simulink library "pathFollowingExp_LAS"  (R2020a)
settings: Solver=VariableStepAuto  StartTime=0.0  StopTime=10.0  RelTol=1e-3
undefined symbols (not defined in the file or in its folder): fltCtrl, pathCtrl, vhcl
libraries: pathFollowingControllerExp_cl x4, courseFollowExp_cl x1, ctrlAllocMatrix_cl x1
settings Model: Creator=jcreed2  LastModifiedBy=jcreed2

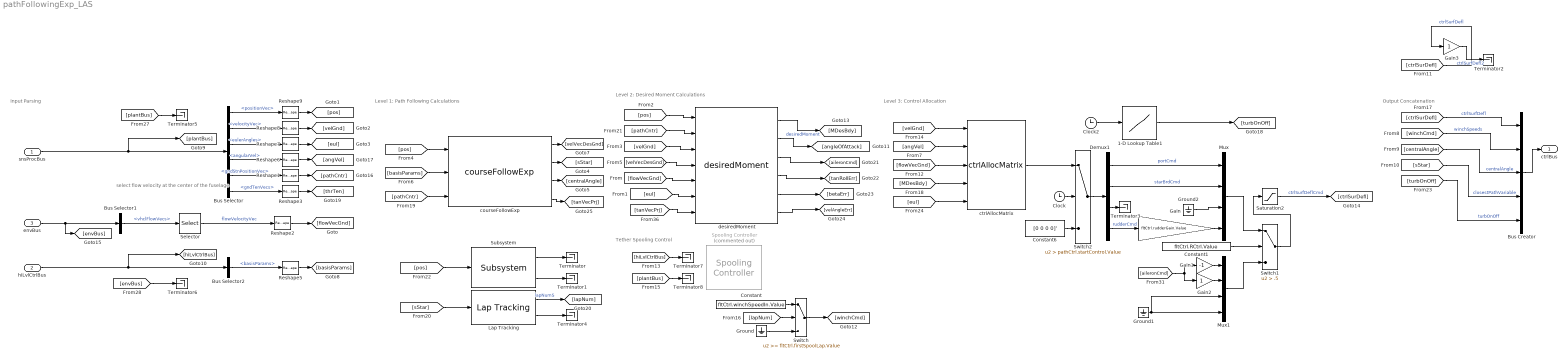
== system pathFollowingExp_LAS ==
  note: Output Concatenation
  note: Level 2: Desired Moment Calculations
  note: Input Parsing
  note: Level 1: Path Following Calculations
  note: Tether Spooling Control
  note: select flow velocity at the center of the fuselage
  note: Level 3: Control Allocation
  snsProcBus : Inport  OutDataTypeStr=Bus: sensorsProcessingBus
  hiLvlCtrlBus : Inport  Port=2  OutDataTypeStr=Bus: hiLvlCtrlBus
  envBus : Inport  Port=3  OutDataTypeStr=Bus: envBus
  1-D Lookup Table1 : Lookup_n-D  NumberOfTableDimensions=1  BreakpointsForDimension1=[0 1000 2000]  Table=[0 0 0]  InterpMethod=Flat  InternalRulePriority=Speed  RndMeth=Simplest  InputSameDT=on
  Bus Creator : BusCreator  Inputs=5  OutDataTypeStr=Bus: fltCtrlBus
      settings: InheritFromInputs=off
  Bus Selector : BusSelector  OutputSignals=positionVec,velocityVec,eulerAngles,angularVel,gndStnPositionVec,gndTenVecs
  Bus Selector1 : BusSelector  OutputSignals=vhclFlowVecs
  Bus Selector2 : BusSelector  OutputSignals=basisParams
  Clock : Clock
  Clock2 : Clock
  Constant : Constant  Value=fltCtrl.winchSpeedIn.Value
  Constant1 : Constant  Value=fltCtrl.RCtrl.Value
  Constant6 : Constant  Value=[0 0 0 0]'
  Demux1 : Demux
  Gain : Gain  Gain=fltCtrl.rudderGain.Value
  Gain1 : Gain  Gain=-1
  Gain2 : Gain
  Gain3 : Gain
  Ground : Ground
  Ground1 : Ground
  Ground2 : Ground
  Lap Tracking : pathFollowingControllerExp_cl/pathFollowingControllerExp/Lap Tracking  SystemSampleTime=-1  Latency=0  AutoFrameSizeCalculation=off
  Mux : Mux
  Mux1 : Mux
  Reshape{1..3,5..9} (8 alike) : Reshape  OutputDimensionality=Column vector (2-D)
  Saturation2 : Saturate  UpperLimit=pathCtrl.controlSigMax.upperLimit.Value  LowerLimit=pathCtrl.controlSigMax.lowerLimit.Value
  Selector : Selector  NumberOfDimensions=2  InputPortWidth=3  IndexOptions=Select all,Index vector (dialog)  Indices=[1 3],5  OutputSizes=1,1
  "Spooling Controller " : pathFollowingControllerExp_cl/pathFollowingControllerExp/Spooling Controller   Commented=on  SystemSampleTime=-1  Latency=0  AutoFrameSizeCalculation=off
  Subsystem : pathFollowingControllerExp_cl/pathFollowingControllerExp/Subsystem  SystemSampleTime=-1  Latency=0  AutoFrameSizeCalculation=off
  Switch : Switch  Threshold=fltCtrl.firstSpoolLap.Value
  Switch1 : Switch  Criteria=u2 > Threshold  Threshold=.5
  Switch2 : Switch  Criteria=u2 > Threshold  Threshold=pathCtrl.startControl.Value
  Terminator{,1..8} (9 alike) : Terminator
  courseFollowExp : courseFollowExp_cl/courseFollowExp  SystemSampleTime=-1  Latency=0  AutoFrameSizeCalculation=off
  ctrlAllocMatrix : ctrlAllocMatrix_cl/ctrlAllocMatrix  aeroStruct=vhcl.struct('OCT.aeroSurf')  fluidDensity=fluidDensity
  desiredMoment : pathFollowingControllerExp_cl/pathFollowingControllerExp/desiredMoment  SystemSampleTime=-1  Latency=0  AutoFrameSizeCalculation=off
  ctrlBus : Outport  OutDataTypeStr=Bus: fltCtrlBus  VectorParamsAs1DForOutWhenUnconnected=off
  wires:
  Bus Selector/6 -> Reshape3/1  "<gndTenVecs>"
  snsProcBus/1 -> [plantBus], Bus Selector/1
  Demux1/1 -> Mux/1  "portCmd"
  [pos] -> courseFollowExp/1
  Demux1/2 -> Mux/2  "starBrdCmd"
  hiLvlCtrlBus/1 -> Bus Selector2/1, [hiLvlCtrlBus]
  Saturation2/1 -> [ctrlSurDefl]  "ctrlSurfDeflCmd"
  Constant/1 -> Switch/1
  Switch1/1 -> Saturation2/1
  courseFollowExp/3 -> [centralAngle]
  Bus Selector/2 -> Reshape8/1  "<velocityVec>"
  [velGnd] -> ctrlAllocMatrix/1
  Bus Selector/3 -> Reshape7/1  "<eulerAngles>"
  Bus Selector1/1 -> Selector/1  "<vhclFlowVecs>"
  Bus Selector/1 -> Reshape9/1  "<positionVec>"
  Lap Tracking/2 -> Terminator4/1
  [pos] -> desiredMoment/1
  Reshape3/1 -> [thrTen]
  envBus/1 -> Bus Selector1/1, [envBus]
  courseFollowExp/1 -> [velVecDesGnd]
  Demux1/4 -> Gain/1  "rudderCmd"
  Bus Creator/1 -> ctrlBus/1
  [winchCmd] -> Bus Creator/2  "winchSpeeds"
  [turbOnOff] -> Bus Creator/5  "turbOnOff"
  courseFollowExp/4 -> [tanVecPrj]
  courseFollowExp/2 -> [sStar]
  Selector/1 -> Reshape2/1  "flowVelocityVec"
  [centralAngle] -> Bus Creator/3  "centralAngle"
  desiredMoment/1 -> [MDesBdy]  "desiredMoment"
  [tanVecPrj] -> desiredMoment/7
  [sStar] -> Bus Creator/4  "closestPathVariable"
  [flowVecGnd] -> ctrlAllocMatrix/3
  [eul] -> desiredMoment/6
  [ctrlSurDefl] -> Gain3/1  "ctrlSurfDefl"
  [ctrlSurDefl] -> Bus Creator/1  "ctrlSurfDefl"
  [pathCntr] -> courseFollowExp/3
  [MDesBdy] -> ctrlAllocMatrix/4
  Constant6/1 -> Switch2/3
  Bus Selector/4 -> Reshape6/1  "<angularVel>"
  Switch2/1 -> Demux1/1
  Reshape6/1 -> [angVel]
  Bus Selector/5 -> Reshape1/1  "<gndStnPositionVec>"
  [pathCntr] -> desiredMoment/2
  Constant1/1 -> Switch1/2
  [flowVecGnd] -> desiredMoment/5
  ctrlAllocMatrix/1 -> Switch2/1
  Reshape2/1 -> [flowVecGnd]
  Reshape8/1 -> [velGnd]
  Reshape1/1 -> [pathCntr]
  [velGnd] -> desiredMoment/3
  Clock2/1 -> 1-D Lookup Table1/1
  [eul] -> ctrlAllocMatrix/5
  Bus Selector2/1 -> Reshape5/1  "<basisParams>"
  Gain/1 -> Mux/4
  [basisParams] -> courseFollowExp/2
  [pos] -> Subsystem/1
  Reshape9/1 -> [pos]
  desiredMoment/2 -> [angleOfAttack]
  Ground2/1 -> Mux/3
  [plantBus] -> Terminator8/1
  Demux1/3 -> Terminator3/1
  Clock/1 -> Switch2/2
  [plantBus] -> Terminator5/1
  Lap Tracking/1 -> [lapNum]  "lapNumS"
  [hiLvlCtrlBus] -> Terminator7/1
  Reshape7/1 -> [eul]
  Subsystem/1 -> Terminator/1
  Subsystem/2 -> Terminator1/1
  [envBus] -> Terminator6/1
  [sStar] -> Lap Tracking/1
  [velVecDesGnd] -> desiredMoment/4
  desiredMoment/3 -> [aileronCmd]
  [angVel] -> ctrlAllocMatrix/2
  [aileronCmd] -> Gain2/1, Gain1/1
  [lapNum] -> Switch/2
  Ground/1 -> Switch/3
  Gain2/1 -> Mux1/2
  Switch/1 -> [winchCmd]
  1-D Lookup Table1/1 -> [turbOnOff]
  Gain1/1 -> Mux1/1
  desiredMoment/6 -> [velAngleErr]
  Reshape5/1 -> [basisParams]
  Mux1/1 -> Switch1/3
  desiredMoment/5 -> [betaErr]
  Gain3/1 -> Terminator2/1  "ctrlSurfDefl2"
  desiredMoment/4 -> [tanRollErr]
  Ground1/1 -> Mux1/4, Mux1/3
  Mux/1 -> Switch1/1
